simulink model "RBDmodel_unprotected"  (R2023a)
settings: Solver=ode15s  StartTime=0.0  StopTime=10  FixedStep=0.0001  RelTol=1e-3  AbsTol=1e-3  EnableMultiTasking=on
model workspace (MAT data in the model file):
  C_Gimbal = 0.1
  C_IAP = 0.01
  IAP_Pa = 0
  K_Gimbal = 0
  K_IAP = 0
  Left_EO = 0
  Left_IO = 0
  Left_MF = 0
  Left_RA = 0
  Moment_AR = 0
  Moment_FE = 7.5
  Moment_LB = 0
  Right_EO = 0
  Right_IO = 0
  Right_MF = 0
  Right_RA = 0
  a = 1
  b = 1
  muscle_color = [0 0 1]
  muscle_radius = 1
undefined symbols (not defined in the file): X, Y, Z
libraries: nesl_utility x346, sm_lib x329, simulink_extras x33, checkpacklib x3, simulink x1
(part 2 of 13)

== system RBDmodel_unprotected/Right ITL Readings ==
  In1 : Inport
  In2 : Inport  Port=2
  In3 : Inport  Port=3
  In4 : Inport  Port=4
  In5 : Inport  Port=5
  Right L1-L2 ITL force : Scope
  Right L2-L3 ITL force : Scope
  Right L3-L4 ITL force : Scope
  Right L4-L5 ITL force : Scope
  Right L5-S1 ITL force : Scope
  wires:
  In5/1 -> Right L3-L4 ITL force/1
  In3/1 -> Right L5-S1 ITL force/1
  In2/1 -> Right L2-L3 ITL force/1
  In1/1 -> Right L1-L2 ITL force/1
  In4/1 -> Right L4-L5 ITL force/1

== system RBDmodel_unprotected/SSL Readings ==
  In1 : Inport
  In2 : Inport  Port=2
  In3 : Inport  Port=3
  In4 : Inport  Port=4
  In5 : Inport  Port=5
  L1-L2 SSL force : Scope
  L2-L3 SSL force : Scope
  L3-L4 SSL force : Scope
  L4-L5 SSL force : Scope
  L5-S1 SSL force : Scope
  wires:
  In5/1 -> L5-S1 SSL force/1
  In3/1 -> L1-L2 SSL force/1
  In1/1 -> L2-L3 SSL force/1
  In2/1 -> L3-L4 SSL force/1
  In4/1 -> L4-L5 SSL force/1

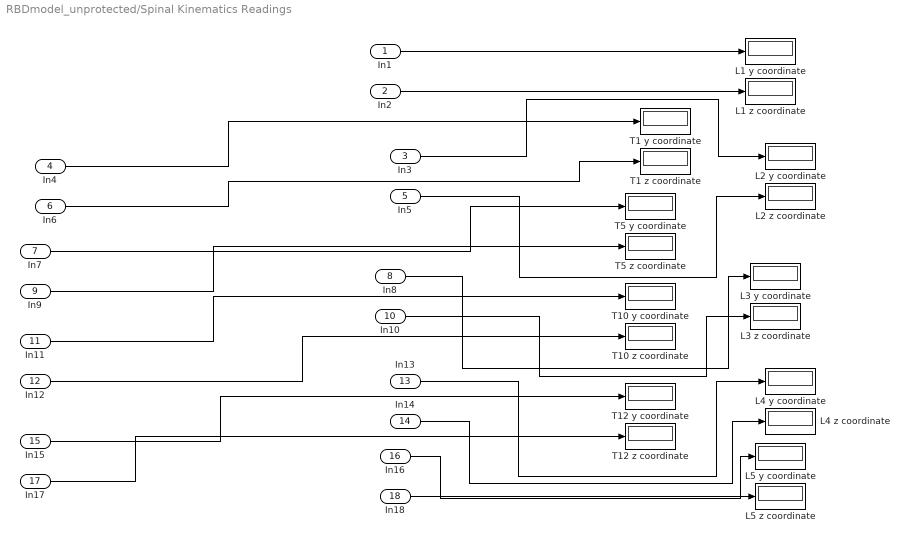
== system RBDmodel_unprotected/Spinal Kinematics Readings ==
  In1 : Inport
  In2 : Inport  Port=2
  In3 : Inport  Port=3
  In4 : Inport  Port=4
  In5 : Inport  Port=5
  In6 : Inport  Port=6
  In7 : Inport  Port=7
  In8 : Inport  Port=8
  In9 : Inport  Port=9
  In10 : Inport  Port=10
  In11 : Inport  Port=11
  In12 : Inport  Port=12
  In13 : Inport  Port=13
  In14 : Inport  Port=14
  In15 : Inport  Port=15
  In16 : Inport  Port=16
  In17 : Inport  Port=17
  In18 : Inport  Port=18
  L1 y coordinate : Display
  L1 z coordinate : Display
  L2 y coordinate : Display
  L2 z coordinate : Display
  L3 y coordinate : Display
  L3 z coordinate : Display
  L4 y coordinate : Display
  L4 z coordinate : Display
  L5 y coordinate : Display
  L5 z coordinate : Display
  T1 y coordinate : Display
  T1 z coordinate : Display
  T10 y coordinate : Display
  T10 z coordinate : Display
  T12 y coordinate : Display
  T12 z coordinate : Display
  T5 y coordinate : Display
  T5 z coordinate : Display
  wires:
  In2/1 -> L1 z coordinate/1
  In7/1 -> T5 y coordinate/1
  In13/1 -> L4 y coordinate/1
  In10/1 -> L3 z coordinate/1
  In18/1 -> L5 z coordinate/1
  In6/1 -> T1 z coordinate/1
  In3/1 -> L2 y coordinate/1
  In11/1 -> T10 y coordinate/1
  In9/1 -> T5 z coordinate/1
  In1/1 -> L1 y coordinate/1
  In5/1 -> L2 z coordinate/1
  In14/1 -> L4 z coordinate/1
  In15/1 -> T12 y coordinate/1
  In4/1 -> T1 y coordinate/1
  In12/1 -> T10 z coordinate/1
  In8/1 -> L3 y coordinate/1
  In17/1 -> T12 z coordinate/1
  In16/1 -> L5 y coordinate/1

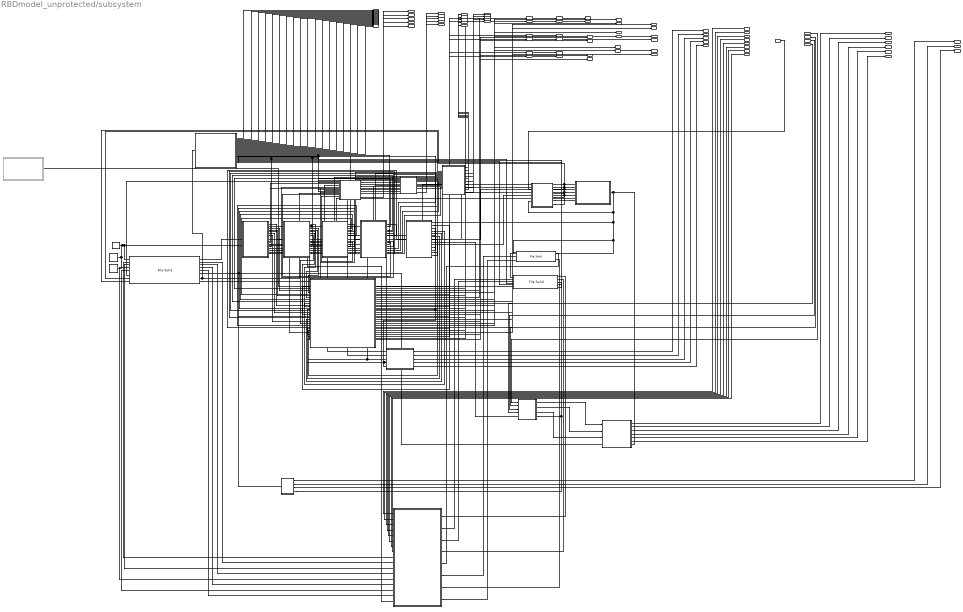
== system RBDmodel_unprotected/subsystem ==
  RightAbdominalMuscleForce : Inport  OutDataTypeStr=double  PortDimensions=1
  LeftAbdominalMuscleForce : Inport  Port=2  OutDataTypeStr=double  PortDimensions=1
  input0 : Inport  Port=3  OutDataTypeStr=double  PortDimensions=1  SampleTime=0
  RightBackMuscleForce : Inport  Port=4  OutDataTypeStr=double  PortDimensions=1
  input1 : Inport  Port=5  OutDataTypeStr=double  PortDimensions=1  SampleTime=0
  LeftBackMuscleForce : Inport  Port=6  OutDataTypeStr=double  PortDimensions=1
  In7 : Inport  Port=7  OutDataTypeStr=double  PortDimensions=1
  input2 : Inport  Port=8  OutDataTypeStr=double  PortDimensions=1  SampleTime=0
  RightTransverse1MuscleForce : Inport  Port=9  OutDataTypeStr=double  PortDimensions=1
  input3 : Inport  Port=10  OutDataTypeStr=double  PortDimensions=1  SampleTime=0
  RightTransverse2MuscleForce : Inport  Port=11  OutDataTypeStr=double  PortDimensions=1
  LeftTransverse1MuscleForce : Inport  Port=12  OutDataTypeStr=double  PortDimensions=1
  LeftTransverse2MuscleForce : Inport  Port=13  OutDataTypeStr=double  PortDimensions=1
  Extensor torque setup : Subsystem
  Hand : Subsystem  Commented=on
  IAP Model 1 setup : Subsystem
  IAP Model 2 setup : Subsystem
  ISL setup : Subsystem
  ITL setup : Subsystem
  L1 : Subsystem
  L1 moment setup : Subsystem
  L1-S1 readings setup : Subsystem
  L2 : Subsystem
  L3 : Subsystem
  L4 : Subsystem
  L5 : Subsystem
  Left T Spine : sm_lib/Body Elements/File Solid  ExtGeomFileName=C:\Users\siril\OneDrive\Desktop\TIM-Control\Matlab\Simscape models\CAD - with COM\SymmetricModel\draft7\LeftThoracicSpineWithRibcage.step  UnitType=FromFile  ExtGeomFileUnits=m  StepReaderType=HEX  ExportConvexHullGeometry=off  InertiaType=CalculateFromGeometry  Mass=1  MassUnits=kg  CenterOfMass=[0 0 0]  CenterOfMassUnits=m  MomentsOfInertia=[1 1 1]  MomentsOfInertiaUnits=kg*m^2  ProductsOfInertia=[0 0 0]  ProductsOfInertiaUnits=kg*m^2  BasedOnType=Density  Density=0.182  DensityUnits=g/cm^3  DoExposeReferenceFrame=off  SerializedFrames=<Frames><Frame><Id>Frame1</Id><Value><Name>To L1</Name><Origin><Source>GeometricFeature</Source><FeatureName>segment 762</FeatureName></Origin><PrimaryAxis><DefinedDirection>-Z</DefinedDirection><Source>GeometricFeature</Source><SourceDirection>+Z</SourceDirection><FeatureName>planar surface 1266</FeatureName></PrimaryAxis><SecondaryAxis><DefinedDirection>+X</DefinedDirection><Source>ReferenceFrame</Source><SourceDirection>+X</SourceDirection><FeatureName></FeatureName></SecondaryAxis></Value></Frame><Frame><Id>Frame2</Id><Value><Name>To Left Abdominal Muscle</Name><Origin><Source>GeometricFeature</Source><FeatureName>planar surface 54556</FeatureName></Origin><PrimaryAxis><DefinedDirection>+Z</DefinedDirection><Source>GeometricFeature</Source><SourceDirection>+Z</SourceDirection><FeatureName>planar surface 54556</FeatureName></PrimaryAxis><SecondaryAxis><DefinedDirection>+X</DefinedDirection><Source>ReferenceFrame</Source><SourceDirection>+X</SourceDirection><FeatureName></FeatureName></SecondaryAxis></Value></Frame><Frame><Id>Frame3</Id><Value><Name>To Left Back Muscle</Name><Origin><Source>GeometricFeature</Source><FeatureName>planar surface 54574</FeatureName></Origin><PrimaryAxis><DefinedDirection>-Z</DefinedDirection><Source>GeometricFeature</Source><SourceDirection>+Z</SourceDirection><FeatureName>planar surface 54574</FeatureName></PrimaryAxis><SecondaryAxis><DefinedDirection>+X</DefinedDirection><Source>ReferenceFrame</Source><SourceDirection>+X</SourceDirection><FeatureName></FeatureName></SecondaryAxis></Value></Frame><Frame><Id>Frame4</Id><Value><Name>To Left Transverse1 Muscle</Name><Origin><Source>GeometricFeature</Source><FeatureName>planar surface 54586</FeatureName></Origin><PrimaryAxis><DefinedDirection>+Z</DefinedDirection><Source>GeometricFeature</Source><SourceDirection>+Z</SourceDirection><FeatureName>planar surface 54586</FeatureName></PrimaryAxis><SecondaryAxis><DefinedDirection>+X</DefinedDirection><Source>ReferenceFrame</Source><SourceDirection>+X</SourceDirection><FeatureName></FeatureName></SecondaryAxis></Value></Frame><Frame><Id>Frame5</Id><Value><Name>To Left Transverse2 Muscle</Name><Origin><Source>GeometricFeature</Source><FeatureName>planar surface 54611</FeatureName></Origin><PrimaryAxis><DefinedDirection>+Z</DefinedDirection><Source>GeometricFeature</Source><SourceDirection>+Z</SourceDirection><FeatureName>planar surface 54611</FeatureName></PrimaryAxis><SecondaryAxis><DefinedDirection>+X</DefinedDirection><Source>ReferenceFrame</Source><SourceDirection>+X</SourceDirection><FeatureName></FeatureName></SecondaryAxis></Value></Frame></Frames>  GraphicType=FromGeometry  MarkerShape=Sphere  MarkerSize=10  GraphicVisPropType=SimpleVisualProperties  GraphicDiffuseColor=[0.8901961 0.8745098 0.7254902]  GraphicSpecularColor=[0.5 0.5 0.5 1.0]  GraphicAmbientColor=[0.15 0.15 0.15 1.0]  GraphicEmissiveColor=[0.0 0.0 0.0 1.0]  GraphicShininess=75  GraphicOpacity=1.0
  Mechanism Configuration : sm_lib/Utilities/Mechanism Configuration  UniformGravity=Constant  GravityVector=[0 0 -9.80665]  GravityVectorUnits=m/s^2  LinearizationDelta=0.001  JointModeTransitionNonlinearIterations=2
  Muscle Forces setup : Subsystem
  Plumbline setup : Subsystem
  Right T Spine : sm_lib/Body Elements/File Solid  ExtGeomFileName=C:\Users\siril\OneDrive\Desktop\TIM-Control\Matlab\Simscape models\CAD - with COM\SymmetricModel\draft7\RightThoracicSpineWithRibcage.step  UnitType=FromFile  ExtGeomFileUnits=m  StepReaderType=HEX  ExportConvexHullGeometry=off  InertiaType=CalculateFromGeometry  Mass=1  MassUnits=kg  CenterOfMass=[0 0 0]  CenterOfMassUnits=m  MomentsOfInertia=[1 1 1]  MomentsOfInertiaUnits=kg*m^2  ProductsOfInertia=[0 0 0]  ProductsOfInertiaUnits=kg*m^2  BasedOnType=Density  Density=0.182  DensityUnits=g/cm^3  DoExposeReferenceFrame=off  SerializedFrames=<Frames><Frame><Id>Frame1</Id><Value><Name>To L1</Name><Origin><Source>GeometricFeature</Source><FeatureName>segment 633</FeatureName></Origin><PrimaryAxis><DefinedDirection>+Z</DefinedDirection><Source>GeometricFeature</Source><SourceDirection>+Z</SourceDirection><FeatureName>planar surface 1266</FeatureName></PrimaryAxis><SecondaryAxis><DefinedDirection>+X</DefinedDirection><Source>ReferenceFrame</Source><SourceDirection>+X</SourceDirection><FeatureName></FeatureName></SecondaryAxis></Value></Frame><Frame><Id>Frame2</Id><Value><Name>To Right Abdominal Muscle</Name><Origin><Source>GeometricFeature</Source><FeatureName>planar surface 54556</FeatureName></Origin><PrimaryAxis><DefinedDirection>-Z</DefinedDirection><Source>GeometricFeature</Source><SourceDirection>+Z</SourceDirection><FeatureName>planar surface 54556</FeatureName></PrimaryAxis><SecondaryAxis><DefinedDirection>+X</DefinedDirection><Source>ReferenceFrame</Source><SourceDirection>+X</SourceDirection><FeatureName></FeatureName></SecondaryAxis></Value></Frame><Frame><Id>Frame3</Id><Value><Name>To Right Back Muscle</Name><Origin><Source>GeometricFeature</Source><FeatureName>planar surface 54574</FeatureName></Origin><PrimaryAxis><DefinedDirection>+Z</DefinedDirection><Source>GeometricFeature</Source><SourceDirection>+Z</SourceDirection><FeatureName>planar surface 54574</FeatureName></PrimaryAxis><SecondaryAxis><DefinedDirection>+X</DefinedDirection><Source>ReferenceFrame</Source><SourceDirection>+X</SourceDirection><FeatureName></FeatureName></SecondaryAxis></Value></Frame><Frame><Id>Frame4</Id><Value><Name>To Right Transverse1 Muscle</Name><Origin><Source>GeometricFeature</Source><FeatureName>planar surface 54586</FeatureName></Origin><PrimaryAxis><DefinedDirection>-Z</DefinedDirection><Source>GeometricFeature</Source><SourceDirection>+Z</SourceDirection><FeatureName>planar surface 54586</FeatureName></PrimaryAxis><SecondaryAxis><DefinedDirection>+X</DefinedDirection><Source>ReferenceFrame</Source><SourceDirection>+X</SourceDirection><FeatureName></FeatureName></SecondaryAxis></Value></Frame><Frame><Id>Frame5</Id><Value><Name>To Right Transverse2 Muscle</Name><Origin><Source>GeometricFeature</Source><FeatureName>planar surface 54611</FeatureName></Origin><PrimaryAxis><DefinedDirection>-Z</DefinedDirection><Source>GeometricFeature</Source><SourceDirection>+Z</SourceDirection><FeatureName>planar surface 54611</FeatureName></PrimaryAxis><SecondaryAxis><DefinedDirection>+X</DefinedDirection><Source>ReferenceFrame</Source><SourceDirection>+X</SourceDirection><FeatureName></FeatureName></SecondaryAxis></Value></Frame><Frame><Id>Frame6</Id><Value><Name>T1 Plumbline Frame</Name><Origin><Source>GeometricFeature</Source><FeatureName>point 5793</FeatureName></Origin><PrimaryAxis><DefinedDirection>+Z</DefinedDirection><Source>ReferenceFrame</Source><SourceDirection>+Z</SourceDirection><FeatureName></FeatureName></PrimaryAxis><SecondaryAxis><DefinedDirection>+X</DefinedDirection><Source>ReferenceFrame</Source><SourceDirection>+X</SourceDirection><FeatureName></FeatureName></SecondaryAxis></Value></Frame><Frame><Id>Frame7</Id><Value><Name>T5 Spinous Process Tip</Name><Origin><Source>GeometricFeature</Source><FeatureName>point 6426</FeatureName></Origin><PrimaryAxis><DefinedDirection>+Z</DefinedDirection><Source>ReferenceFrame</Source><SourceDirection>+Z</SourceDirection><FeatureName></FeatureName></PrimaryAxis><SecondaryAxis><DefinedDirection>+X</DefinedDirection><Source>ReferenceFrame</Source><SourceDirection>+X</SourceDirection><FeatureName></FeatureName></SecondaryAxis></Value></Frame><Frame><Id>Frame8</Id><Value><Name>T1 Spinous Process Tip</Name><Origin><Source>GeometricFeature</Source><FeatureName>point 327</FeatureName></Origin><PrimaryAxis><DefinedDirection>+Z</DefinedDirection><Source>ReferenceFrame</Source><SourceDirection>+Z</SourceDirection><FeatureName></FeatureName></PrimaryAxis><SecondaryAxis><DefinedDirection>+X</DefinedDirection><Source>ReferenceFrame</Source><SourceDirection>+X</SourceDirection><FeatureName></FeatureName></SecondaryAxis></Value></Frame><Frame><Id>Frame9</Id><Value><Name>T10 Spinous process tip</Name><Origin><Source>GeometricFeature</Source><FeatureName>point 46212</FeatureName></Origin><PrimaryAxis><DefinedDirection>+Z</DefinedDirection><Source>ReferenceFrame</Source><SourceDirection>+Z</SourceDirection><FeatureName></FeatureName></PrimaryAxis><SecondaryAxis><DefinedDirection>+X</DefinedDirection><Source>ReferenceFrame</Source><SourceDirection>+X</SourceDirection><FeatureName></FeatureName></SecondaryAxis></Value></Frame><Frame><Id>Frame10</Id><Value><Name>T12 Spinous Process tip</Name><Origin><Source>GeometricFeature</Source><FeatureName>point 4338</FeatureName></Origin><PrimaryAxis><DefinedDirection>+Z</DefinedDirection><Source>ReferenceFrame</Source><SourceDirection>+Z</SourceDirection><FeatureName></FeatureName></PrimaryAxis><SecondaryAxis><DefinedDirection>+X</DefinedDirection><Source>ReferenceFrame</Source><SourceDirection>+X</SourceDirection><FeatureName></FeatureName></SecondaryAxis></Value></Frame><Frame><Id>Frame11</Id><Value><Name>To Clavicle</Name><Origin><Source>GeometricFeature</Source><FeatureName>point 134734</FeatureName></Origin><PrimaryAxis><DefinedDirection>+Z</DefinedDirection><Source>ReferenceFrame</Source><SourceDirection>+Z</SourceDirection><FeatureName></FeatureName></PrimaryAxis><SecondaryAxis><DefinedDirection>+X</DefinedDirection><Source>ReferenceFrame</Source><SourceDirection>+X</SourceDirection><FeatureName></FeatureName></SecondaryAxis></Value></Frame></Frames>  GraphicType=FromGeometry  MarkerShape=Sphere  MarkerSize=10  GraphicVisPropType=SimpleVisualProperties  GraphicDiffuseColor=[0.8901961 0.8745098 0.7254902]  GraphicSpecularColor=[0.5 0.5 0.5 1.0]  GraphicAmbientColor=[0.15 0.15 0.15 1.0]  GraphicEmissiveColor=[0.0 0.0 0.0 1.0]  GraphicShininess=75  GraphicOpacity=1.0
  SSL Setup : Subsystem
  Segmental Moment-Rotation setup : Subsystem
  Solver Configuration : nesl_utility/Solver Configuration  PhysicalDomain=network_engine_domain  SubClassName=solver  LeftPortType=input  RightPortType=generic  Tones=[]  Harmonics=[]  SimulateNoise=off  Profile=off  UseLocalSampling=off  EnableSwitchedLinearOptims=on  FrequencyDomain=off  UseCCode=off  RelTol=0.001  AbsTol=1e-06  MinStep=1e-09  ToWorkspace=off  RevertToSquareIcSolve=off  NumHomotopyIterations=100  PhasorMode=off  PhasorModeNumHarmonics=1  ConsistencySolver=NEWTON_FTOL  IndexReductionMethod=DerivativeReplacement  DoDC=off  ResidualTolerance=1e-09  ConsistencyTolSource=GLOBAL  ConsistencyAbsTol=0.001  ConsistencyRelTol=0.001  ConsistencyTolFactor=0.001  UseLocalSolver=off  LocalSolverChoice=NE_BACKWARD_EULER_ADVANCER  ResolveIndetEquations=on  FunctionEvalNumThread=1  LocalSolverSampleTime=0.001  DoFixedCost=off  MaxNonlinIter=3  MaxModeIter=2  ComputeImpulses=off  ImpulseIterations=2  LinearAlgebra=Sparse  LinearAlgebraNumThread=0  EquationFormulation=NE_TIME_EF  DelaysMemoryBudget=1024  AutomaticFiltering=on  FilteringTimeConstant=0.001  PartitionStorageMethod=AS_NEEDED  PartitionMemoryBudget=1024  PartitionMethod=FAST
  Spinal Kinematics Setup : Subsystem
  World Frame : sm_lib/Frames and Transforms/World Frame
  sacrum : sm_lib/Body Elements/File Solid  ExtGeomFileName=C:\Users\siril\OneDrive\Desktop\TIM-Control\Matlab\Simscape models\CAD - with COM\SymmetricModel\sacrum.step  UnitType=FromFile  ExtGeomFileUnits=m  StepReaderType=HEX  ExportConvexHullGeometry=off  InertiaType=CalculateFromGeometry  Mass=1  MassUnits=kg  CenterOfMass=[0 0 0]  CenterOfMassUnits=m  MomentsOfInertia=[1 1 1]  MomentsOfInertiaUnits=kg*m^2  ProductsOfInertia=[0 0 0]  ProductsOfInertiaUnits=kg*m^2  BasedOnType=Density  Density=0.182  DensityUnits=g/cm^3  DoExposeReferenceFrame=on  SerializedFrames=<Frames><Frame><Id>Frame1</Id><Value><Name>To L5</Name><Origin><Source>GeometricFeature</Source><FeatureName>planar surface 14566</FeatureName></Origin><PrimaryAxis><DefinedDirection>+Z</DefinedDirection><Source>GeometricFeature</Source><SourceDirection>+Z</SourceDirection><FeatureName>planar surface 14566</FeatureName></PrimaryAxis><SecondaryAxis><DefinedDirection>+X</DefinedDirection><Source>ReferenceFrame</Source><SourceDirection>+X</SourceDirection><FeatureName></FeatureName></SecondaryAxis></Value></Frame><Frame><Id>Frame2</Id><Value><Name>To Right Abdominal Muscle</Name><Origin><Source>GeometricFeature</Source><FeatureName>planar surface 54</FeatureName></Origin><PrimaryAxis><DefinedDirection>+Z</DefinedDirection><Source>ReferenceFrame</Source><SourceDirection>+Z</SourceDirection><FeatureName></FeatureName></PrimaryAxis><SecondaryAxis><DefinedDirection>+X</DefinedDirection><Source>ReferenceFrame</Source><SourceDirection>+X</SourceDirection><FeatureName></FeatureName></SecondaryAxis></Value></Frame><Frame><Id>Frame3</Id><Value><Name>To Left Abdominal Muscle</Name><Origin><Source>GeometricFeature</Source><FeatureName>planar surface 7390</FeatureName></Origin><PrimaryAxis><DefinedDirection>+Z</DefinedDirection><Source>ReferenceFrame</Source><SourceDirection>+Z</SourceDirection><FeatureName></FeatureName></PrimaryAxis><SecondaryAxis><DefinedDirection>+X</DefinedDirection><Source>ReferenceFrame</Source><SourceDirection>+X</SourceDirection><FeatureName></FeatureName></SecondaryAxis></Value></Frame><Frame><Id>Frame4</Id><Value><Name>To Right Back Muscle</Name><Origin><Source>GeometricFeature</Source><FeatureName>planar surface 26</FeatureName></Origin><PrimaryAxis><DefinedDirection>+Z</DefinedDirection><Source>ReferenceFrame</Source><SourceDirection>+Z</SourceDirection><FeatureName></FeatureName></PrimaryAxis><SecondaryAxis><DefinedDirection>+X</DefinedDirection><Source>ReferenceFrame</Source><SourceDirection>+X</SourceDirection><FeatureName></FeatureName></SecondaryAxis></Value></Frame><Frame><Id>Frame5</Id><Value><Name>To Left Back Muscle</Name><Origin><Source>GeometricFeature</Source><FeatureName>planar surface 7362</FeatureName></Origin><PrimaryAxis><DefinedDirection>+Z</DefinedDirection><Source>ReferenceFrame</Source><SourceDirection>+Z</SourceDirection><FeatureName></FeatureName></PrimaryAxis><SecondaryAxis><DefinedDirection>+X</DefinedDirection><Source>ReferenceFrame</Source><SourceDirection>+X</SourceDirection><FeatureName></FeatureName></SecondaryAxis></Value></Frame><Frame><Id>Frame6</Id><Value><Name>To Right Transverse1 Muscle</Name><Origin><Source>GeometricFeature</Source><FeatureName>planar surface 19</FeatureName></Origin><PrimaryAxis><DefinedDirection>+Z</DefinedDirection><Source>ReferenceFrame</Source><SourceDirection>+Z</SourceDirection><FeatureName></FeatureName></PrimaryAxis><SecondaryAxis><DefinedDirection>+X</DefinedDirection><Source>ReferenceFrame</Source><SourceDirection>+X</SourceDirection><FeatureName></FeatureName></SecondaryAxis></Value></Frame><Frame><Id>Frame7</Id><Value><Name>To Right Transverse2 Muscle</Name><Origin><Source>GeometricFeature</Source><FeatureName>planar surface 5</FeatureName></Origin><PrimaryAxis><DefinedDirection>+Z</DefinedDirection><Source>ReferenceFrame</Source><SourceDirection>+Z</SourceDirection><FeatureName></FeatureName></PrimaryAxis><SecondaryAxis><DefinedDirection>+X</DefinedDirection><Source>ReferenceFrame</Source><SourceDirection>+X</SourceDirection><FeatureName></FeatureName></SecondaryAxis></Value></Frame><Frame><Id>Frame8</Id><Value><Name>To Left Transverse1 Muscle</Name><Origin><Source>GeometricFeature</Source><FeatureName>planar surface 7355</FeatureName></Origin><PrimaryAxis><DefinedDirection>+Z</DefinedDirection><Source>ReferenceFrame</Source><SourceDirection>+Z</SourceDirection><FeatureName></FeatureName></PrimaryAxis><SecondaryAxis><DefinedDirection>+X</DefinedDirection><Source>ReferenceFrame</Source><SourceDirection>+X</SourceDirection><FeatureName></FeatureName></SecondaryAxis></Value></Frame><Frame><Id>Frame9</Id><Value><Name>To Left Transverse2 Muscle</Name><Origin><Source>GeometricFeature</Source><FeatureName>planar surface 7341</FeatureName></Origin><PrimaryAxis><DefinedDirection>+Z</DefinedDirection><Source>ReferenceFrame</Source><SourceDirection>+Z</SourceDirection><FeatureName></FeatureName></PrimaryAxis><SecondaryAxis><DefinedDirection>+X</DefinedDirection><Source>ReferenceFrame</Source><SourceDirection>+X</SourceDirection><FeatureName></FeatureName></SecondaryAxis></Value></Frame><Frame><Id>Frame10</Id><Value><Name>For Plumbline Evaluation</Name><Origin><Source>GeometricFeature</Source><FeatureName>planar surface 14546</FeatureName></Origin><PrimaryAxis><DefinedDirection>+Z</DefinedDirection><Source>ReferenceFrame</Source><SourceDirection>+Z</SourceDirection><FeatureName></FeatureName></PrimaryAxis><SecondaryAxis><DefinedDirection>+X</DefinedDirection><Source>ReferenceFrame</Source><SourceDirection>+X</SourceDirection><FeatureName></FeatureName></SecondaryAxis></Value></Frame><Frame><Id>Frame11</Id><Value><Name>To Abdomen - Right</Name><Origin><Source>GeometricFeature</Source><FeatureName>planar surface 2380</FeatureName></Origin><PrimaryAxis><DefinedDirection>+Z</DefinedDirection><Source>ReferenceFrame</Source><SourceDirection>+Z</SourceDirection><FeatureName></FeatureName></PrimaryAxis><SecondaryAxis><DefinedDirection>+X</DefinedDirection><Source>ReferenceFrame</Source><SourceDirection>+X</SourceDirection><FeatureName></FeatureName></SecondaryAxis></Value></Frame><Frame><Id>Frame12</Id><Value><Name>To Abdomen - Left</Name><Origin><Source>GeometricFeature</Source><FeatureName>planar surface 9716</FeatureName></Origin><PrimaryAxis><DefinedDirection>+Z</DefinedDirection><Source>ReferenceFrame</Source><SourceDirection>+Z</SourceDirection><FeatureName></FeatureName></PrimaryAxis><SecondaryAxis><DefinedDirection>+X</DefinedDirection><Source>ReferenceFrame</Source><SourceDirection>+X</SourceDirection><FeatureName></FeatureName></SecondaryAxis></Value></Frame><Frame><Id>Frame13</Id><Value><Name>To L5 ISL</Name><Origin><Source>GeometricFeature</Source><FeatureName>point 22330</FeatureName></Origin><PrimaryAxis><DefinedDirection>+Z</DefinedDirection><Source>ReferenceFrame</Source><SourceDirection>+Z</SourceDirection><FeatureName></FeatureName></PrimaryAxis><SecondaryAxis><DefinedDirection>+X</DefinedDirection><Source>ReferenceFrame</Source><SourceDirection>+X</SourceDirection><FeatureName></FeatureName></SecondaryAxis></Value></Frame><Frame><Id>Frame14</Id><Value><Name>To L5 SSL</Name><Origin><Source>GeometricFeature</Source><FeatureName>point 44660</FeatureName></Origin><PrimaryAxis><DefinedDirection>+Z</DefinedDirection><Source>ReferenceFrame</Source><SourceDirection>+Z</SourceDirection><FeatureName></FeatureName></PrimaryAxis><SecondaryAxis><DefinedDirection>+X</DefinedDirection><Source>ReferenceFrame</Source><SourceDirection>+X</SourceDirection><FeatureName></FeatureName></SecondaryAxis></Value></Frame><Frame><Id>Frame15</Id><Value><Name>To Right L5 ITL</Name><Origin><Source>GeometricFeature</Source><FeatureName>point 13718</FeatureName></Origin><PrimaryAxis><DefinedDirection>+Z</DefinedDirection><Source>ReferenceFrame</Source><SourceDirection>+Z</SourceDirection><FeatureName></FeatureName></PrimaryAxis><SecondaryAxis><DefinedDirection>+X</DefinedDirection><Source>ReferenceFrame</Source><SourceDirection>+X</SourceDirection><FeatureName></FeatureName></SecondaryAxis></Value></Frame><Frame><Id>Frame16</Id><Value><Name>To left L5 ITL</Name><Origin><Source>GeometricFeature</Source><FeatureName>point 36305</FeatureName></Origin><PrimaryAxis><DefinedDirection>+Z</DefinedDirection><Source>ReferenceFrame</Source><SourceDirection>+Z</SourceDirection><FeatureName></FeatureName></PrimaryAxis><SecondaryAxis><DefinedDirection>+X</DefinedDirection><Source>ReferenceFrame</Source><SourceDirection>+X</SourceDirection><FeatureName></FeatureName></SecondaryAxis></Value></Frame><Frame><Id>Frame17</Id><Value><Name>Sacrum COM</Name><Origin><Source>CenterOfMassFrame</Source><FeatureName></FeatureName></Origin><PrimaryAxis><DefinedDirection>+Z</DefinedDirection><Source>ReferenceFrame</Source><SourceDirection>+Z</SourceDirection><FeatureName></FeatureName></PrimaryAxis><SecondaryAxis><DefinedDirection>+X</DefinedDirection><Source>ReferenceFrame</Source><SourceDirection>+X</SourceDirection><FeatureName></FeatureName></SecondaryAxis></Value></Frame></Frames>  GraphicType=FromGeometry  MarkerShape=Sphere  MarkerSize=10  GraphicVisPropType=SimpleVisualProperties  GraphicDiffuseColor=[0.8901961 0.8509804 0.6117647]  GraphicSpecularColor=[0.5 0.5 0.5 1.0]  GraphicAmbientColor=[0.15 0.15 0.15 1.0]  GraphicEmissiveColor=[0.0 0.0 0.0 1.0]  GraphicShininess=75  GraphicOpacity=1.0
  Out1 : Outport  OutDataTypeStr=double  PortDimensions=[1 1]  SampleTime=0
  Out2 : Outport  Port=2  OutDataTypeStr=double  PortDimensions=[1 1]  SampleTime=0
  Out3 : Outport  Port=3  OutDataTypeStr=double  PortDimensions=[1 1]  SampleTime=0
  Out4 : Outport  Port=4  OutDataTypeStr=double  PortDimensions=[1 1]  SampleTime=0
  Out5 : Outport  Port=5  OutDataTypeStr=double  PortDimensions=[1 1]  SampleTime=0
  Out6 : Outport  Port=6  OutDataTypeStr=double  PortDimensions=[1 1]  SampleTime=0
  Out7 : Outport  Port=7  OutDataTypeStr=double  PortDimensions=[1 1]  SampleTime=0
  Out8 : Outport  Port=8  OutDataTypeStr=double  PortDimensions=[1 1]  SampleTime=0
  Out9 : Outport  Port=9  OutDataTypeStr=double  PortDimensions=[1 1]  SampleTime=0
  Out10 : Outport  Port=10  OutDataTypeStr=double  PortDimensions=[1 1]  SampleTime=0
  Out11 : Outport  Port=11  OutDataTypeStr=double  PortDimensions=[1 1]  SampleTime=0
  Out12 : Outport  Port=12  OutDataTypeStr=double  PortDimensions=[1 1]  SampleTime=0
  Out13 : Outport  Port=13  OutDataTypeStr=double  PortDimensions=[1 1]  SampleTime=0
  Out14 : Outport  Port=14  OutDataTypeStr=double  PortDimensions=[1 1]  SampleTime=0
  Out15 : Outport  Port=15  OutDataTypeStr=double  PortDimensions=[1 1]  SampleTime=0
  Out16 : Outport  Port=16  OutDataTypeStr=double  PortDimensions=[1 1]  SampleTime=0
  Out17 : Outport  Port=17  OutDataTypeStr=double  PortDimensions=[1 1]  SampleTime=0
  Out18 : Outport  Port=18  OutDataTypeStr=double  PortDimensions=[1 1]  SampleTime=0
  L5-S1 FE Simscape Rotation : Outport  Port=19  OutDataTypeStr=double  PortDimensions=1  SampleTime=0
  L4-L5 FE Simscape Rotation : Outport  Port=20  OutDataTypeStr=double  PortDimensions=1  SampleTime=0
  L3-L4 FE Simscape Rotation : Outport  Port=21  OutDataTypeStr=double  PortDimensions=1  SampleTime=0
  Out22 : Outport  Port=22  OutDataTypeStr=double  PortDimensions=[1 1]  SampleTime=0
  Out23 : Outport  Port=23  OutDataTypeStr=double  PortDimensions=[1 1]  SampleTime=0
  Out24 : Outport  Port=24  OutDataTypeStr=double  PortDimensions=[1 1]  SampleTime=0
  Out25 : Outport  Port=25  OutDataTypeStr=double  PortDimensions=[1 1]  SampleTime=0
  Out26 : Outport  Port=26  OutDataTypeStr=double  PortDimensions=[1 1]  SampleTime=0
  Out27 : Outport  Port=27  OutDataTypeStr=double  PortDimensions=[1 1]  SampleTime=0
  L2-L3 FE Simscape Rotation : Outport  Port=28  OutDataTypeStr=double  PortDimensions=1  SampleTime=0
  Out29 : Outport  Port=29  OutDataTypeStr=double  PortDimensions=[1 1]  SampleTime=0
  Out30 : Outport  Port=30  OutDataTypeStr=double  PortDimensions=[1 1]  SampleTime=0
  Out31 : Outport  Port=31  OutDataTypeStr=double  PortDimensions=[1 1]  SampleTime=0
  Out32 : Outport  Port=32  OutDataTypeStr=double  PortDimensions=[1 1]  SampleTime=0
  L5-S1 FE Simscape Moment : Outport  Port=33  OutDataTypeStr=double  PortDimensions=1  SampleTime=0
  L4-L5 FE Simscape Moment : Outport  Port=34  OutDataTypeStr=double  PortDimensions=1  SampleTime=0
  L3-L4 FE Simscape Moment : Outport  Port=35  OutDataTypeStr=double  PortDimensions=1  SampleTime=0
  Out36 : Outport  Port=36  OutDataTypeStr=double  PortDimensions=[1 1]  SampleTime=0
  Out37 : Outport  Port=37  OutDataTypeStr=double  PortDimensions=[1 1]  SampleTime=0
  Out38 : Outport  Port=38  OutDataTypeStr=double  PortDimensions=[1 1]  SampleTime=0
  Out39 : Outport  Port=39  OutDataTypeStr=double  PortDimensions=[1 1]  SampleTime=0
  L2-L3 FE Simscape Moment : Outport  Port=40  OutDataTypeStr=double  PortDimensions=1  SampleTime=0
  Out41 : Outport  Port=41  OutDataTypeStr=double  PortDimensions=[1 1]  SampleTime=0
  Out42 : Outport  Port=42  OutDataTypeStr=double  PortDimensions=[1 1]  SampleTime=0
  L1-L2 FE Simscape Rotation : Outport  Port=43  OutDataTypeStr=double  PortDimensions=1  SampleTime=0
  Out44 : Outport  Port=44  OutDataTypeStr=double  PortDimensions=[1 1]  SampleTime=0
  Out45 : Outport  Port=45  OutDataTypeStr=double  PortDimensions=[1 1]  SampleTime=0
  Out46 : Outport  Port=46  OutDataTypeStr=double  PortDimensions=[1 1]  SampleTime=0
  Out47 : Outport  Port=47  OutDataTypeStr=double  PortDimensions=[1 1]  SampleTime=0
  L1-L2 FE Simscape Moment : Outport  Port=48  OutDataTypeStr=double  PortDimensions=1  SampleTime=0
  output : Outport  Port=49  OutDataTypeStr=double  PortDimensions=[1 1]  SampleTime=0
  L2-L3 LB Simscape Rotation : Outport  Port=50  OutDataTypeStr=double  PortDimensions=1  SampleTime=0
  L1-S1 FE Simscape Rotation : Outport  Port=51  OutDataTypeStr=double  PortDimensions=[1 1]  SampleTime=0
  Out52 : Outport  Port=52  OutDataTypeStr=double  PortDimensions=[1 1]  SampleTime=0
  L5-S1 LB Simscape Rotation : Outport  Port=53  OutDataTypeStr=double  PortDimensions=1  SampleTime=0
  L4-L5 LB Simscape Rotation : Outport  Port=54  OutDataTypeStr=double  PortDimensions=1  SampleTime=0
  L2-L3 LB Simscape Moment : Outport  Port=55  OutDataTypeStr=double  PortDimensions=1  SampleTime=0
  L1-L2 LB Simscape Rotation : Outport  Port=56  OutDataTypeStr=double  PortDimensions=1  SampleTime=0
  L3-L4 LB Simscape Rotation : Outport  Port=57  OutDataTypeStr=double  PortDimensions=1  SampleTime=0
  Out58 : Outport  Port=58  OutDataTypeStr=double  PortDimensions=[1 1]  SampleTime=0
  L1-S1 FE Simscape Moment : Outport  Port=59  OutDataTypeStr=double  PortDimensions=1  SampleTime=0
  L5-S1 LB Simscape Moment : Outport  Port=60  OutDataTypeStr=double  PortDimensions=1  SampleTime=0
  L4-L5 LB Simscape Moment : Outport  Port=61  OutDataTypeStr=double  PortDimensions=1  SampleTime=0
  L1-L2 LB Simscape Moment : Outport  Port=62  OutDataTypeStr=double  PortDimensions=1  SampleTime=0
  L3-L4 LB Simscape Moment : Outport  Port=63  OutDataTypeStr=double  PortDimensions=1  SampleTime=0
  Out64 : Outport  Port=64  OutDataTypeStr=double  PortDimensions=[1 1]  SampleTime=0
  x : Outport  Port=65  OutDataTypeStr=double  PortDimensions=[1 1]  SampleTime=0
  L1-S1 LB Simscape Rotation : Outport  Port=66  OutDataTypeStr=double  PortDimensions=[1 1]  SampleTime=0
  Out67 : Outport  Port=67  OutDataTypeStr=double  PortDimensions=[1 1]  SampleTime=0
  y : Outport  Port=68  OutDataTypeStr=double  PortDimensions=[1 1]  SampleTime=0
  L2-L3 AR Simscape Rotation : Outport  Port=69  OutDataTypeStr=double  PortDimensions=1  SampleTime=0
  L1-S1 LB Simscape Moment : Outport  Port=70  OutDataTypeStr=double  PortDimensions=1  SampleTime=0
  L2-L3 AR Simscape Moment : Outport  Port=71  OutDataTypeStr=double  PortDimensions=1  SampleTime=0
  L1-L2 AR Simscape Rotation : Outport  Port=72  OutDataTypeStr=double  PortDimensions=1  SampleTime=0
  z : Outport  Port=73  OutDataTypeStr=double  PortDimensions=[1 1]  SampleTime=0
  L1-S1 AR Simscape Rotation : Outport  Port=74  OutDataTypeStr=double  PortDimensions=[1 1]  SampleTime=0
  L5-S1 AR Simscape Rotation : Outport  Port=75  OutDataTypeStr=double  PortDimensions=1  SampleTime=0
  L4-L5 AR Simscape Rotation : Outport  Port=76  OutDataTypeStr=double  PortDimensions=1  SampleTime=0
  L1-L2 AR Simscape Moment : Outport  Port=77  OutDataTypeStr=double  PortDimensions=1  SampleTime=0
  L3-L4 AR Simscape Rotation : Outport  Port=78  OutDataTypeStr=double  PortDimensions=1  SampleTime=0
  L5-S1 AR Simscape Moment : Outport  Port=79  OutDataTypeStr=double  PortDimensions=1  SampleTime=0
  L4-L5 AR Simscape Moment : Outport  Port=80  OutDataTypeStr=double  PortDimensions=1  SampleTime=0
  L1-S1 AR Simscape Moment : Outport  Port=81  OutDataTypeStr=double  PortDimensions=1  SampleTime=0
  L3-L4 AR Simscape Moment : Outport  Port=82  OutDataTypeStr=double  PortDimensions=1  SampleTime=0
  wires:
  ISL setup/5(Out5) -> Out47/1
  Segmental Moment-Rotation setup/10(L1-L2 FE Simscape Moment) -> L1-L2 FE Simscape Moment/1  "L1-L2 FE Simscape Moment"
  ITL setup/2(Out2) -> Out16/1
  input0/1 -> L1 moment setup/1(input0)
  Plumbline setup/2(y) -> y/1  "y"
  ISL setup/3(Out3) -> Out23/1
  RightTransverse1MuscleForce/1 -> Muscle Forces setup/5(RightTransverse1MuscleForce)  "RightTransverse1MuscleForce"
  ITL setup/3(Out3) -> Out9/1
  Segmental Moment-Rotation setup/12(L5-S1 LB Simscape Rotation) -> L5-S1 LB Simscape Rotation/1  "L5-S1 LB Simscape Rotation"
  L1 moment setup/3(Out3) -> L1-S1 readings setup/3(In3)
  SSL Setup/4(Out4) -> Out31/1
  Segmental Moment-Rotation setup/30(L3-L4 AR Simscape Moment) -> L3-L4 AR Simscape Moment/1  "L3-L4 AR Simscape Moment"
  Spinal Kinematics Setup/7(Out7) -> Out12/1
  Extensor torque setup/2(Out2) -> Out52/1
  RightAbdominalMuscleForce/1 -> Muscle Forces setup/1(RightAbdominalMuscleForce)  "RightAbdominalMuscleForce"
  Segmental Moment-Rotation setup/2(L4-L5 FE Simscape Rotation) -> L4-L5 FE Simscape Rotation/1  "L4-L5 FE Simscape Rotation"
  L1-S1 readings setup/6(L1-S1 AR Simscape Moment) -> L1-S1 AR Simscape Moment/1  "L1-S1 AR Simscape Moment"
  ISL setup/1(Out1) -> Out3/1
  SSL Setup/3(Out3) -> Out24/1
  ITL setup/5(Out5) -> Out26/1
  Extensor torque setup/5(Out5) -> Out67/1
  Segmental Moment-Rotation setup/8(L2-L3 FE Simscape Moment) -> L2-L3 FE Simscape Moment/1  "L2-L3 FE Simscape Moment"
  L1 moment setup/1(Out1) -> L1-S1 readings setup/1(In1)
  L1 moment setup/2(Out2) -> L1-S1 readings setup/2(In2)
  Segmental Moment-Rotation setup/25(L4-L5 AR Simscape Rotation) -> L4-L5 AR Simscape Rotation/1  "L4-L5 AR Simscape Rotation"
  L1-S1 readings setup/4(L1-S1 LB Simscape Moment) -> L1-S1 LB Simscape Moment/1  "L1-S1 LB Simscape Moment"
  LeftTransverse2MuscleForce/1 -> Muscle Forces setup/8(LeftTransverse2MuscleForce)  "LeftTransverse2MuscleForce"
  Segmental Moment-Rotation setup/29(L4-L5 AR Simscape Moment) -> L4-L5 AR Simscape Moment/1  "L4-L5 AR Simscape Moment"
  Spinal Kinematics Setup/5(Out5) -> Out7/1
  Spinal Kinematics Setup/17(Out17) -> Out44/1
  Segmental Moment-Rotation setup/15(L1-L2 LB Simscape Rotation) -> L1-L2 LB Simscape Rotation/1  "L1-L2 LB Simscape Rotation"
  Segmental Moment-Rotation setup/13(L4-L5 LB Simscape Rotation) -> L4-L5 LB Simscape Rotation/1  "L4-L5 LB Simscape Rotation"
  Segmental Moment-Rotation setup/7(L3-L4 FE Simscape Moment) -> L3-L4 FE Simscape Moment/1  "L3-L4 FE Simscape Moment"
  L1-S1 readings setup/2(L1-S1 FE Simscape Moment) -> L1-S1 FE Simscape Moment/1  "L1-S1 FE Simscape Moment"
  Extensor torque setup/3(Out3) -> Out58/1
  Segmental Moment-Rotation setup/26(L1-L2 AR Simscape Moment) -> L1-L2 AR Simscape Moment/1  "L1-L2 AR Simscape Moment"
  Extensor torque setup/4(Out4) -> Out64/1
  Segmental Moment-Rotation setup/22(L2-L3 AR Simscape Moment) -> L2-L3 AR Simscape Moment/1  "L2-L3 AR Simscape Moment"
  Extensor torque setup/1(output) -> output/1
  ISL setup/4(Out4) -> Out37/1
  L1-S1 readings setup/3(L1-S1 LB Simscape Rotation) -> L1-S1 LB Simscape Rotation/1  "L1-S1 LB Simscape Rotation"
  LeftTransverse1MuscleForce/1 -> Muscle Forces setup/7(LeftTransverse1MuscleForce)  "LeftTransverse1MuscleForce"
  LeftBackMuscleForce/1 -> Muscle Forces setup/4(LeftBackMuscleForce)  "LeftBackMuscleForce"
  RightBackMuscleForce/1 -> Muscle Forces setup/3(RightBackMuscleForce)  "RightBackMuscleForce"
  RightTransverse2MuscleForce/1 -> Muscle Forces setup/6(RightTransverse2MuscleForce)  "RightTransverse2MuscleForce"
  Spinal Kinematics Setup/10(Out10) -> Out22/1
  LeftAbdominalMuscleForce/1 -> Muscle Forces setup/2(LeftAbdominalMuscleForce)  "LeftAbdominalMuscleForce"
  In7/1 -> IAP Model 1 setup/1(In1)
  Segmental Moment-Rotation setup/28(L5-S1 AR Simscape Moment) -> L5-S1 AR Simscape Moment/1  "L5-S1 AR Simscape Moment"
  Segmental Moment-Rotation setup/27(L3-L4 AR Simscape Rotation) -> L3-L4 AR Simscape Rotation/1  "L3-L4 AR Simscape Rotation"
  Segmental Moment-Rotation setup/1(L5-S1 FE Simscape Rotation) -> L5-S1 FE Simscape Rotation/1  "L5-S1 FE Simscape Rotation"
  Plumbline setup/1(x) -> x/1  "x"
  Spinal Kinematics Setup/18(Out18) -> Out46/1
  Plumbline setup/3(z) -> z/1  "z"
  Segmental Moment-Rotation setup/23(L1-L2 AR Simscape Rotation) -> L1-L2 AR Simscape Rotation/1  "L1-L2 AR Simscape Rotation"
  Segmental Moment-Rotation setup/24(L5-S1 AR Simscape Rotation) -> L5-S1 AR Simscape Rotation/1  "L5-S1 AR Simscape Rotation"
  Segmental Moment-Rotation setup/19(L1-L2 LB Simscape Moment) -> L1-L2 LB Simscape Moment/1  "L1-L2 LB Simscape Moment"
  Segmental Moment-Rotation setup/20(L3-L4 LB Simscape Moment) -> L3-L4 LB Simscape Moment/1  "L3-L4 LB Simscape Moment"
  Segmental Moment-Rotation setup/21(L2-L3 AR Simscape Rotation) -> L2-L3 AR Simscape Rotation/1  "L2-L3 AR Simscape Rotation"
  Spinal Kinematics Setup/12(Out12) -> Out29/1
  ITL setup/10(Out10) -> Out32/1
  Spinal Kinematics Setup/8(Out8) -> Out15/1
  Spinal Kinematics Setup/11(Out11) -> Out25/1
  Spinal Kinematics Setup/4(Out4) -> Out5/1
  Spinal Kinematics Setup/2(Out2) -> Out2/1
  Segmental Moment-Rotation setup/9(L1-L2 FE Simscape Rotation) -> L1-L2 FE Simscape Rotation/1  "L1-L2 FE Simscape Rotation"
  Spinal Kinematics Setup/6(Out6) -> Out10/1
  Spinal Kinematics Setup/3(Out3) -> Out4/1
  Spinal Kinematics Setup/1(Out1) -> Out1/1
  L1-S1 readings setup/5(L1-S1 AR Simscape Rotation) -> L1-S1 AR Simscape Rotation/1  "L1-S1 AR Simscape Rotation"
  Spinal Kinematics Setup/9(Out9) -> Out17/1
  Spinal Kinematics Setup/13(Out13) -> Out30/1
  Spinal Kinematics Setup/14(Out14) -> Out36/1
  input2/1 -> L1 moment setup/3(input2)
  Spinal Kinematics Setup/16(Out16) -> Out41/1
  Spinal Kinematics Setup/15(Out15) -> Out39/1
  L1-S1 readings setup/1(L1-S1 FE Simscape Rotation) -> L1-S1 FE Simscape Rotation/1  "L1-S1 FE Simscape Rotation"
  ISL setup/2(Out2) -> Out11/1
  ITL setup/1(Out1) -> Out8/1
  Segmental Moment-Rotation setup/11(L2-L3 LB Simscape Rotation) -> L2-L3 LB Simscape Rotation/1  "L2-L3 LB Simscape Rotation"
  Segmental Moment-Rotation setup/16(L3-L4 LB Simscape Rotation) -> L3-L4 LB Simscape Rotation/1  "L3-L4 LB Simscape Rotation"
  ITL setup/4(Out4) -> Out14/1
  ITL setup/6(Out6) -> Out18/1
  ITL setup/7(Out7) -> Out38/1
  Segmental Moment-Rotation setup/14(L2-L3 LB Simscape Moment) -> L2-L3 LB Simscape Moment/1  "L2-L3 LB Simscape Moment"
  ITL setup/9(Out9) -> Out45/1
  ITL setup/8(Out8) -> Out27/1
  Segmental Moment-Rotation setup/17(L5-S1 LB Simscape Moment) -> L5-S1 LB Simscape Moment/1  "L5-S1 LB Simscape Moment"
  Segmental Moment-Rotation setup/18(L4-L5 LB Simscape Moment) -> L4-L5 LB Simscape Moment/1  "L4-L5 LB Simscape Moment"
  Segmental Moment-Rotation setup/3(L3-L4 FE Simscape Rotation) -> L3-L4 FE Simscape Rotation/1  "L3-L4 FE Simscape Rotation"
  Segmental Moment-Rotation setup/4(L2-L3 FE Simscape Rotation) -> L2-L3 FE Simscape Rotation/1  "L2-L3 FE Simscape Rotation"
  Segmental Moment-Rotation setup/6(L4-L5 FE Simscape Moment) -> L4-L5 FE Simscape Moment/1  "L4-L5 FE Simscape Moment"
  Segmental Moment-Rotation setup/5(L5-S1 FE Simscape Moment) -> L5-S1 FE Simscape Moment/1  "L5-S1 FE Simscape Moment"
  SSL Setup/2(Out2) -> Out13/1
  SSL Setup/1(Out1) -> Out6/1
  SSL Setup/5(Out5) -> Out42/1
  input3/1 -> L1 moment setup/4(input3)
  input1/1 -> L1 moment setup/2(input1)
  connections:
  IAP Model 2 setup/RConn6 -- World Frame/RConn1 -- Mechanism Configuration/RConn1 -- Solver Configuration/RConn1 -- sacrum/RConn1 -- Muscle Forces setup/LConn9
  IAP Model 2 setup/RConn4 -- IAP Model 1 setup/RConn4 -- L3/RConn9
  Right T Spine/RConn3 -- Plumbline setup/RConn1 -- L1 moment setup/RConn1
  sacrum/LConn8 -- SSL Setup/LConn10 -- Spinal Kinematics Setup/LConn1
  Extensor torque setup/LConn4 -- Segmental Moment-Rotation setup/LConn30 -- L2/RConn3
  Spinal Kinematics Setup/RConn4 -- SSL Setup/LConn2 -- L4/RConn12
  IAP Model 2 setup/RConn1 -- IAP Model 1 setup/RConn2 -- L5/RConn9
  IAP Model 2 setup/RConn3 -- IAP Model 1 setup/RConn5 -- L2/RConn9
  sacrum/LConn6 -- Plumbline setup/LConn1 -- L1-S1 readings setup/LConn1
  Extensor torque setup/LConn3 -- Segmental Moment-Rotation setup/LConn28 -- L3/RConn2
  IAP Model 2 setup/LConn1 -- Right T Spine/LConn1 -- Left T Spine/LConn1 -- L1/RConn1 -- IAP Model 1 setup/LConn1 -- L1-S1 readings setup/RConn1
  Spinal Kinematics Setup/RConn5 -- L5/RConn13 -- SSL Setup/LConn4
  L5/RConn2 -- Extensor torque setup/LConn1 -- Segmental Moment-Rotation setup/LConn26
  Spinal Kinematics Setup/RConn1 -- SSL Setup/LConn3 -- L2/RConn12
  Spinal Kinematics Setup/RConn2 -- SSL Setup/LConn8 -- L3/RConn13
  IAP Model 2 setup/RConn2 -- IAP Model 1 setup/RConn3 -- L4/RConn9
  L1/RConn3 -- Extensor torque setup/LConn5 -- Segmental Moment-Rotation setup/LConn27
  IAP Model 2 setup/RConn5 -- IAP Model 1 setup/RConn6 -- L1/RConn9
  Extensor torque setup/LConn2 -- Segmental Moment-Rotation setup/LConn29 -- L4/RConn2
  Spinal Kinematics Setup/RConn3 -- SSL Setup/LConn9 -- L1/RConn11
  L1/RConn2 -- Segmental Moment-Rotation setup/LConn1
  L4/RConn5 -- Segmental Moment-Rotation setup/LConn12
  L3/RConn7 -- Segmental Moment-Rotation setup/LConn22
  IAP Model 2 setup/RConn7 -- sacrum/RConn9
  sacrum/LConn2 -- Muscle Forces setup/LConn2
  L5/RConn16 -- ITL setup/LConn10
  Right T Spine/LConn6 -- Hand/RConn1
  Muscle Forces setup/RConn8 -- Left T Spine/LConn3
  Muscle Forces setup/RConn4 -- Right T Spine/RConn2
  Muscle Forces setup/RConn1 -- Right T Spine/RConn1
  L4/RConn17 -- ITL setup/LConn16
  L3/RConn3 -- Segmental Moment-Rotation setup/LConn5
  L2/RConn1 -- L1/LConn1
  L5/RConn3 -- Segmental Moment-Rotation setup/LConn3
  L1/RConn12 -- ITL setup/LConn14
  Muscle Forces setup/RConn7 -- Left T Spine/RConn2
  L2/RConn4 -- Segmental Moment-Rotation setup/LConn9
  L4/RConn7 -- Segmental Moment-Rotation setup/LConn21
  L5/RConn17 -- ITL setup/LConn15
  Spinal Kinematics Setup/RConn7 -- Right T Spine/RConn4
  sacrum/RConn5 -- Muscle Forces setup/LConn7
  Muscle Forces setup/RConn2 -- Right T Spine/LConn2
  L3/RConn15 -- ITL setup/LConn8
  sacrum/LConn1 -- L5/LConn1
  Spinal Kinematics Setup/RConn9 -- Right T Spine/RConn5
  L1/RConn8 -- L1 moment setup/LConn1
  L3/LConn1 -- L4/RConn1
  Spinal Kinematics Setup/RConn8 -- Right T Spine/LConn5
  Muscle Forces setup/RConn3 -- Right T Spine/LConn3
  L5/RConn4 -- Segmental Moment-Rotation setup/LConn6
  L4/RConn13 -- SSL Setup/LConn5
  Spinal Kinematics Setup/RConn6 -- Right T Spine/LConn4
  L1/RConn6 -- Segmental Moment-Rotation setup/LConn24
  sacrum/RConn4 -- Muscle Forces setup/LConn5
  L3/RConn1 -- L2/LConn1
  L5/RConn1 -- L4/LConn1
  Muscle Forces setup/RConn6 -- Left T Spine/LConn2
  L3/RConn6 -- Segmental Moment-Rotation setup/LConn17
  sacrum/LConn3 -- Muscle Forces setup/LConn4
  Muscle Forces setup/RConn5 -- Left T Spine/RConn1
  L4/RConn3 -- Segmental Moment-Rotation setup/LConn4
  L3/RConn4 -- Segmental Moment-Rotation setup/LConn8
  sacrum/LConn5 -- Muscle Forces setup/LConn8
  sacrum/LConn4 -- Muscle Forces setup/LConn6
  sacrum/RConn3 -- Muscle Forces setup/LConn3
  sacrum/RConn2 -- Muscle Forces setup/LConn1
  L1/RConn7 -- Segmental Moment-Rotation setup/LConn25
  L5/RConn11 -- ISL setup/LConn5
  L1/RConn4 -- Segmental Moment-Rotation setup/LConn10
  L5/RConn5 -- Segmental Moment-Rotation setup/LConn11
  L2/RConn2 -- Segmental Moment-Rotation setup/LConn2
  L3/RConn5 -- Segmental Moment-Rotation setup/LConn13
  L4/RConn15 -- ITL setup/LConn7
  L4/RConn4 -- Segmental Moment-Rotation setup/LConn7
  L4/RConn10 -- ISL setup/LConn3
  L5/RConn10 -- ISL setup/LConn2
  L3/RConn10 -- ISL setup/LConn7
  L3/RConn11 -- ISL setup/LConn9
  L4/RConn11 -- ISL setup/LConn6
  L2/RConn10 -- ISL setup/LConn4
  L1/RConn10 -- ISL setup/LConn10
  L2/RConn11 -- ISL setup/LConn8
  sacrum/RConn7 -- ISL setup/LConn1
  L1/RConn13 -- ITL setup/LConn19
  L2/RConn15 -- ITL setup/LConn9
  L2/RConn17 -- ITL setup/LConn18
  sacrum/LConn9 -- ITL setup/LConn20
  L3/RConn17 -- ITL setup/LConn17
  L3/RConn16 -- ITL setup/LConn12
  L2/RConn16 -- ITL setup/LConn13
  L4/RConn16 -- ITL setup/LConn11
  L5/RConn7 -- Segmental Moment-Rotation setup/LConn20
  L5/RConn14 -- ITL setup/LConn2
  L3/RConn14 -- ITL setup/LConn4
  L4/RConn14 -- ITL setup/LConn3
  L5/RConn15 -- ITL setup/LConn6
  L2/RConn14 -- ITL setup/LConn5
  ITL setup/LConn1 -- sacrum/RConn8
  L3/RConn12 -- SSL Setup/LConn6
  L2/RConn13 -- SSL Setup/LConn7
  L5/RConn12 -- SSL Setup/LConn1
  L2/RConn5 -- Segmental Moment-Rotation setup/LConn14
  L4/RConn6 -- Segmental Moment-Rotation setup/LConn16
  L5/RConn6 -- Segmental Moment-Rotation setup/LConn15
  L1/RConn5 -- Segmental Moment-Rotation setup/LConn19
  L2/RConn6 -- Segmental Moment-Rotation setup/LConn18
  L2/RConn7 -- Segmental Moment-Rotation setup/LConn23

== system RBDmodel_unprotected/subsystem/Extensor torque setup ==
  Add3 : Sum
  Add4 : Sum  Inputs=+++
  Add5 : Sum  Inputs=++++
  Add6 : Sum  Inputs=+++++
  PS-Simulink Converter{6..8,10..21} (15 alike) : nesl_utility/PS-Simulink Converter  PhysicalDomain=network_engine_domain  SubClassName=ps_output  LeftPortType=input  RightPortType=output  PseudoPeriodic=off  Frequencies=[]  VectorFormat=inherit  Unit=inherit  AffineConversion=off
  L5-S1 FE Moment : PMIOPort  Side=Left
  L4-L5 FE Moment : PMIOPort  Port=2  Side=Left
  L3-L4 FE Moment : PMIOPort  Port=3  Side=Left
  L2-L3 FE Moment : PMIOPort  Port=4  Side=Left
  L1-L2 FE Moment : PMIOPort  Port=5  Side=Left
  output : Outport
  Out2 : Outport  Port=2
  Out3 : Outport  Port=3
  Out4 : Outport  Port=4
  Out5 : Outport  Port=5
  wires:
  PS-Simulink Converter16/1 -> Add5/4
  PS-Simulink Converter8/1 -> Add3/2
  PS-Simulink Converter11/1 -> Add4/2
  PS-Simulink Converter7/1 -> Add4/1
  PS-Simulink Converter21/1 -> Add6/5
  PS-Simulink Converter13/1 -> Add5/2
  PS-Simulink Converter12/1 -> Add4/3
  PS-Simulink Converter18/1 -> Add6/3
  Add5/1 -> Out4/1
  Add4/1 -> Out3/1
  PS-Simulink Converter15/1 -> Add5/1
  Add3/1 -> Out2/1
  PS-Simulink Converter10/1 -> Add3/1
  PS-Simulink Converter19/1 -> Add6/1
  PS-Simulink Converter20/1 -> Add6/4
  PS-Simulink Converter17/1 -> Add6/2
  PS-Simulink Converter14/1 -> Add5/3
  PS-Simulink Converter6/1 -> output/1
  Add6/1 -> Out5/1
  connections:
  PS-Simulink Converter20/LConn1 -- PS-Simulink Converter16/LConn1 -- L4-L5 FE Moment/RConn1
  PS-Simulink Converter8/LConn1 -- PS-Simulink Converter17/LConn1 -- PS-Simulink Converter13/LConn1 -- PS-Simulink Converter11/LConn1 -- L2-L3 FE Moment/RConn1
  PS-Simulink Converter18/LConn1 -- PS-Simulink Converter14/LConn1 -- PS-Simulink Converter12/LConn1 -- L3-L4 FE Moment/RConn1
  PS-Simulink Converter10/LConn1 -- PS-Simulink Converter6/LConn1 -- PS-Simulink Converter19/LConn1 -- PS-Simulink Converter15/LConn1 -- PS-Simulink Converter7/LConn1 -- L1-L2 FE Moment/RConn1
  PS-Simulink Converter21/LConn1 -- L5-S1 FE Moment/RConn1
